simulink model "FullDuplex_UDP"  (R2017a)
settings: Solver=FixedStepDiscrete  StartTime=0.0  StopTime=10.0  FixedStep=0.0002  RelTol=1e-3
libraries: stellaris_lp_lib x20, simulink x4, xpcutilitieslib x2, dspswit3 x2
settings Model: ExtModeTrigDuration=8  Creator=peselnikmg  LastModifiedBy=Rorro
settings DataIOCC: LimitDataPoints=on  SaveFormat=Array  SignalLoggingSaveFormat=ModelDataLogs  ReturnWorkspaceOutputs=on
settings OptimizationCC: UseDivisionForNetSlopeComputation=on  UseFloatMulNetSlope=on  DefaultUnderspecifiedDataType=single  UseSpecifiedMinMax=on  PassReuseOutputArgsAs=Individual arguments  ExpressionDepthLimit=2147483647  ZeroExternalMemoryAtStartup=off  NoFixptDivByZeroProtection=on  EfficientFloat2IntCast=on  LifeSpan=inf  MaxStackSize=64  OptimizeBlockOrder=speed
settings DebuggingCC: ReadBeforeWriteMsg=DisableAll  WriteAfterWriteMsg=DisableAll  WriteAfterReadMsg=DisableAll  MultiTaskDSMMsg=none  IntegerOverflowMsg=error  ParameterTunabilityLossMsg=error  AssertControl=DisableAll  StateNameClashWarn=warning  NonBusSignalsTreatedAsBus=error  SFInvalidInputDataAccessInChartInitDiag=error  SFTransitionOutsideNaturalParentDiag=error  SFUnreachableExecutionPathDiag=error  SFUndirectedBroadcastEventsDiag=error  SFExecutionAtInitializationDiag=none  IntegerSaturationMsg=error
settings HardwareCC: ProdBitPerPointer=32  ProdBitPerSizeT=32  ProdBitPerPtrDiffT=32  ProdLargestAtomicInteger=Long  ProdLargestAtomicFloat=Double  ProdWordSize=32  ProdHWDeviceType=ARM Compatible->ARM Cortex
settings ModelReferenceCC: UpdateModelReferenceTargets=IfOutOfDate  PropagateSignalLabelsOutOfModel=off
settings SFSimCC: SFSimEcho=off  MATLABDynamicMemAlloc=off
settings RTWCC: SystemTargetFile=ert.tlc  HardwareBoard=Tiva TM4C123G Launchpad  TLCOptions=-aInlineSetEventsForThisBaseRateFcn=TLC_FALSE -aSuppressMultiTaskScheduler=TLC_FALSE -aRateBasedStepFcn=1  TemplateMakefile=ert_default_tmf  Description=Embedded Coder  GenerateReport=on  RTWVerbose=off  Toolchain=Texas Instruments Code Composer Studio (Tiva)  IncludeHyperlinkInReport=on  LaunchReport=on  GenerateTraceInfo=on  GenerateTraceReport=on  GenerateTraceReportSl=on  GenerateTraceReportSf=on  GenerateTraceReportEml=on
settings CodeAppCC: ForceParamTrailComments=on  IgnoreCustomStorageClasses=off  OperatorAnnotations=on  SimulinkDataObjDesc=on  SFDataObjDesc=on  MATLABFcnDesc=on  CustomSymbolStrType=$N$R$M  InsertBlockDesc=on  MATLABSourceComments=on  EnableCustomComments=on  ReqsInCode=on
settings ERTTargetCC: UtilityFuncGeneration=Shared location  CombineSignalStateStructs=on  SuppressErrorStatus=on  SupportNonFinite=off  ParenthesesLevel=Maximum  CastingMode=Standards  EnableSignedLeftShifts=off  EnableSignedRightShifts=off
settings ConfigComp: CovMetricSettings=dw  CovHtmlReporting=on  CovSaveCumulativeToWorkspaceVar=on  CovSaveSingleToWorkspaceVar=on  CovExternalEMLEnable=off

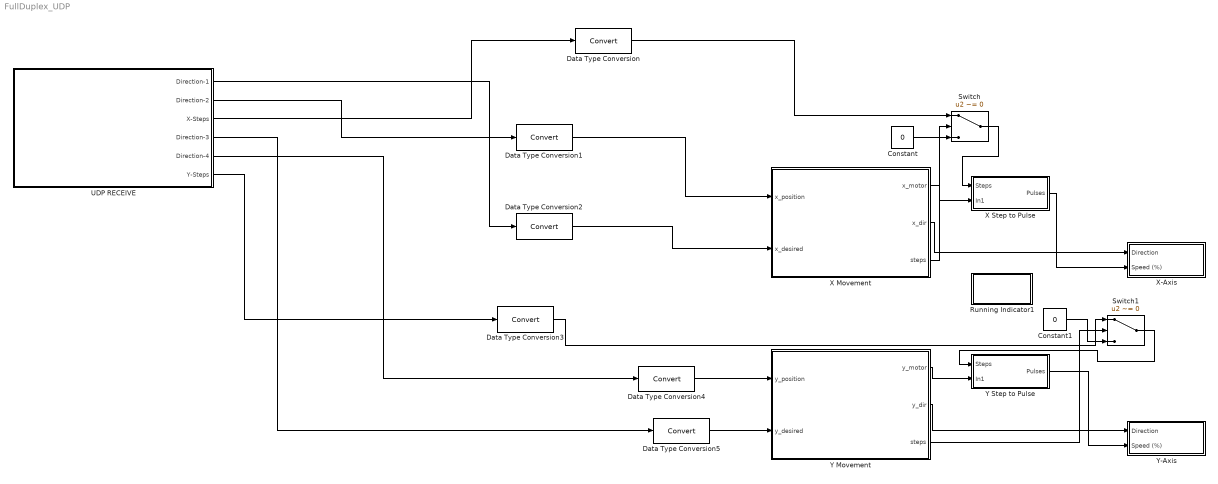
== system FullDuplex_UDP ==
  Constant : Constant  Value=0
  Constant1 : Constant  Value=0
  Data Type Conversion{,1..5} (6 alike) : DataTypeConversion
  Running Indicator1 : Subsystem
  Switch : Switch  Criteria=u2 ~= 0
  Switch1 : Switch  Criteria=u2 ~= 0
  UDP RECEIVE : Subsystem
  X Movement : Stateflow chart  TreatAsAtomicUnit=on
  X Step to Pulse : Subsystem  TreatAsAtomicUnit=on
  X-Axis : Subsystem
  Y Movement : Stateflow chart  TreatAsAtomicUnit=on
  Y Step to Pulse : Subsystem  TreatAsAtomicUnit=on
  Y-Axis : Subsystem
  wires:
  UDP RECEIVE/3(X-Steps) -> Data Type Conversion/1
  Data Type Conversion2/1 -> X Movement/2(x_desired)
  Data Type Conversion1/1 -> X Movement/1(x_position)
  UDP RECEIVE/1("Direction-1 ") -> Data Type Conversion2/1
  UDP RECEIVE/2("Direction-2 ") -> Data Type Conversion1/1
  Y Movement/2(y_dir) -> Y-Axis/1(Direction)
  Y Step to Pulse/1(Pulses) -> Y-Axis/2(Speed (%))
  X Movement/2(x_dir) -> X-Axis/1(Direction)
  Y Movement/1(y_motor) -> Y Step to Pulse/2(In1)
  X Movement/1(x_motor) -> X Step to Pulse/2(In1)
  X Step to Pulse/1(Pulses) -> X-Axis/2(Speed (%))
  UDP RECEIVE/4("Direction-3 ") -> Data Type Conversion5/1
  Data Type Conversion5/1 -> Y Movement/2(y_desired)
  UDP RECEIVE/5("Direction-4 ") -> Data Type Conversion4/1
  Data Type Conversion4/1 -> Y Movement/1(y_position)
  UDP RECEIVE/6(Y-Steps) -> Data Type Conversion3/1
  Data Type Conversion/1 -> Switch/1
  Constant/1 -> Switch/3
  X Movement/3(steps) -> Switch/2
  Switch/1 -> X Step to Pulse/1(Steps)
  Y Movement/3(steps) -> Switch1/2
  Constant1/1 -> Switch1/3
  Switch1/1 -> Y Step to Pulse/1(Steps)
  Data Type Conversion3/1 -> Switch1/1

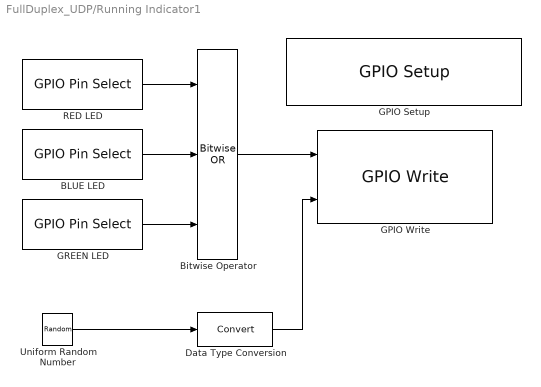
== system FullDuplex_UDP/Running Indicator1 ==
  BLUE LED : stellaris_lp_lib/GPIO/GPIO Pin Select  GPIO_PIN_X=GPIO_PIN_2
      settings: SourceProductName=Run on Stellaris LaunchPad
  Bitwise Operator : simulink/Logic and Bit Operations/Bitwise Operator  logicop=OR  UseBitMask=off  NumInputPorts=3  BitMask=bin2dec('11011001')  BitMaskRealWorld=Stored Integer
  Data Type Conversion : DataTypeConversion
  GPIO Setup : stellaris_lp_lib/GPIO/GPIO Setup  GPIO_PORTX_BASE=GPIO_PORTF_BASE  PinsOutput_0=Input  PinsOutput_1=Output  PinsOutput_2=Output  PinsOutput_3=Output  PinsOutput_4=Input  PinsOutput_5=Input  PinsOutput_6=Input  PinsOutput_7=Input
      settings: SourceProductName=Run on Stellaris LaunchPad
  GPIO Write : stellaris_lp_lib/GPIO/GPIO Write  GPIO_PORTX_BASE=GPIO_PORTF_BASE  SampleTime=-1
      settings: SourceProductName=Run on Stellaris LaunchPad
  GREEN LED : stellaris_lp_lib/GPIO/GPIO Pin Select  GPIO_PIN_X=GPIO_PIN_3
      settings: SourceProductName=Run on Stellaris LaunchPad
  RED LED : stellaris_lp_lib/GPIO/GPIO Pin Select  GPIO_PIN_X=GPIO_PIN_1
      settings: SourceProductName=Run on Stellaris LaunchPad
  Uniform Random Number : UniformRandomNumber  Minimum=0  Maximum=2  SampleTime=0.2
  wires:
  BLUE LED/1 -> Bitwise Operator/2
  RED LED/1 -> Bitwise Operator/1
  GREEN LED/1 -> Bitwise Operator/3
  Bitwise Operator/1 -> GPIO Write/1
  Uniform Random Number/1 -> Data Type Conversion/1
  Data Type Conversion/1 -> GPIO Write/2

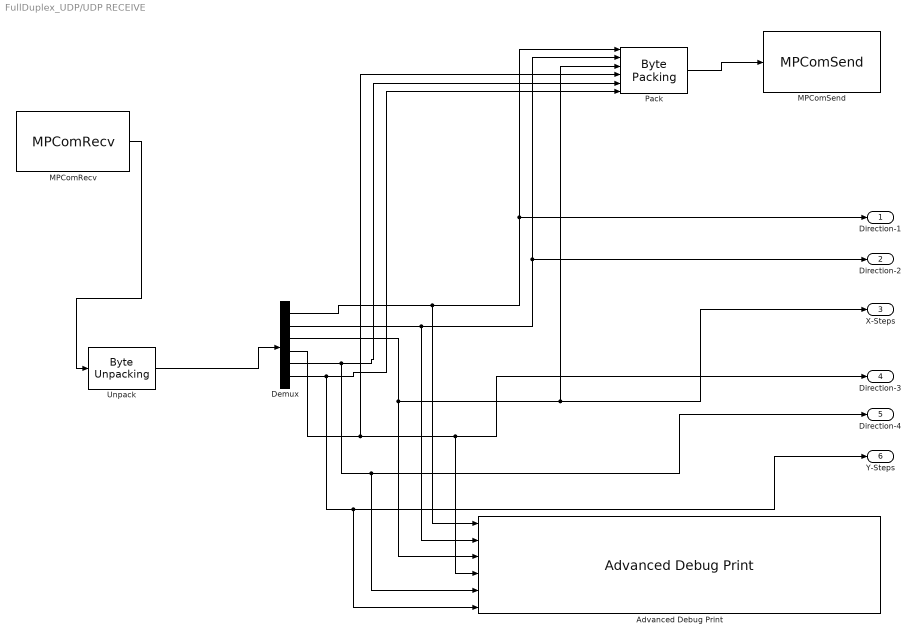
== system FullDuplex_UDP/UDP RECEIVE ==
  Advanced Debug Print : stellaris_lp_lib/Debug/Advanced Debug Print  types={'single','single','single','single','single','single'}  fmt='X: %hf %hf %hf\r\n'  sample_time=1
      settings: SourceProductName=Run on Stellaris LaunchPad
  Demux : Demux  Outputs=6
  MPComRecv : stellaris_lp_lib/Communication/MPComRecv  vport=2  pack_size=24  sample_time=-1
      settings: SourceProductName=Run on Stellaris LaunchPad
  MPComSend : stellaris_lp_lib/Communication/MPComSend  vport=3  pack_size=24  sample_time=-1
      settings: SourceProductName=Run on Stellaris LaunchPad
  Pack : xpcutilitieslib/Byte Packing   MaskPackedDataType=uint8  MaskUnpackedDataTypes={'single','single','single','single','single','single'}  MaskAlignment=1
  Unpack : xpcutilitieslib/Byte Unpacking   MaskUnpackedDataTypes={['single']}  MaskUnpackedDataSizes={[1,6]}  MaskAlignment=1
      settings: SourceProductName=Simulink Real-Time  SourceProductBaseCode=XP
  "Direction-1 " : Outport
  "Direction-2 " : Outport  Port=2
  X-Steps : Outport  Port=3
  "Direction-3 " : Outport  Port=4
  "Direction-4 " : Outport  Port=5
  Y-Steps : Outport  Port=6
  wires:
  Demux/1 -> Advanced Debug Print/1, "Direction-1 "/1, Pack/1
  Demux/2 -> Advanced Debug Print/2, "Direction-2 "/1, Pack/2
  Pack/1 -> MPComSend/1
  MPComRecv/1 -> Unpack/1
  Unpack/1 -> Demux/1
  Demux/3 -> Pack/3, X-Steps/1, Advanced Debug Print/3
  Demux/4 -> "Direction-3 "/1, Advanced Debug Print/4, Pack/4
  Demux/5 -> Pack/5, "Direction-4 "/1, Advanced Debug Print/5
  Demux/6 -> Pack/6, Y-Steps/1, Advanced Debug Print/6

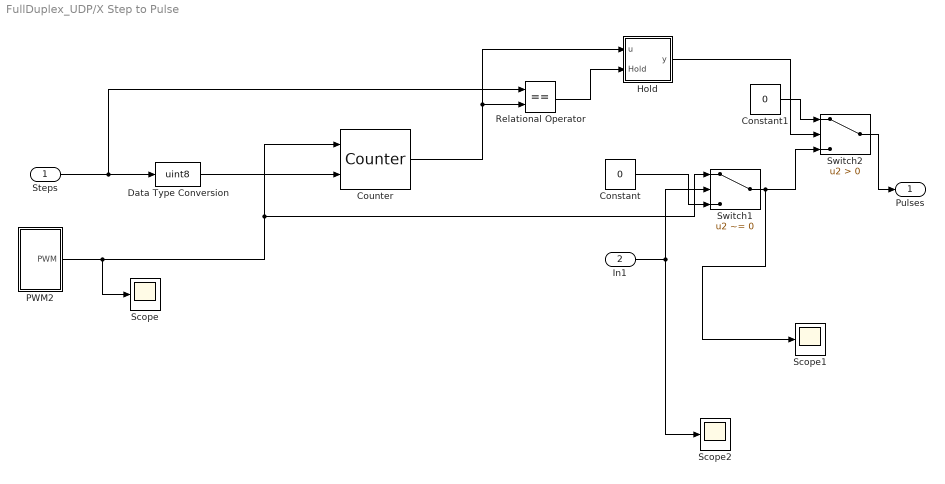
== system FullDuplex_UDP/X Step to Pulse ==
  Steps : Inport
  In1 : Inport  Port=2
  Constant : Constant  Value=0  OutDataTypeStr=single
  Constant1 : Constant  Value=0  OutDataTypeStr=single
  Counter : dspswit3/Counter  Direction=Up  CountEvent=Rising edge  CounterSize=Specify via input port  MaxCount=255  InitialCount=0  Output=Count  HitValue=2  ResetInput=off  SamplesPerFrame=1  Ts=1  CntDtype=single  HitDtype=Logical
  Data Type Conversion : DataTypeConversion  OutDataTypeStr=uint8
  Hold : Subsystem  TreatAsAtomicUnit=on
  PWM2 : Subsystem
  Relational Operator : RelationalOperator  Operator===  OutDataTypeStr=boolean  RndMeth=Simplest
  Scope : Scope
  Scope1 : Scope
  Scope2 : Scope
  Switch1 : Switch  Criteria=u2 ~= 0
  Switch2 : Switch  Criteria=u2 > Threshold
  Pulses : Outport
  wires:
  Steps/1 -> Relational Operator/1, Data Type Conversion/1
  Data Type Conversion/1 -> Counter/2
  Relational Operator/1 -> Hold/2(Hold)
  Switch1/1 -> Scope1/1, Switch2/3
  Counter/1 -> Hold/1(u), Relational Operator/2
  PWM2/1(PWM) -> Scope/1, Switch1/1, Counter/1
  In1/1 -> Scope2/1, Switch1/2
  Constant/1 -> Switch1/3
  Switch2/1 -> Pulses/1
  Constant1/1 -> Switch2/1
  Hold/1(y) -> Switch2/2

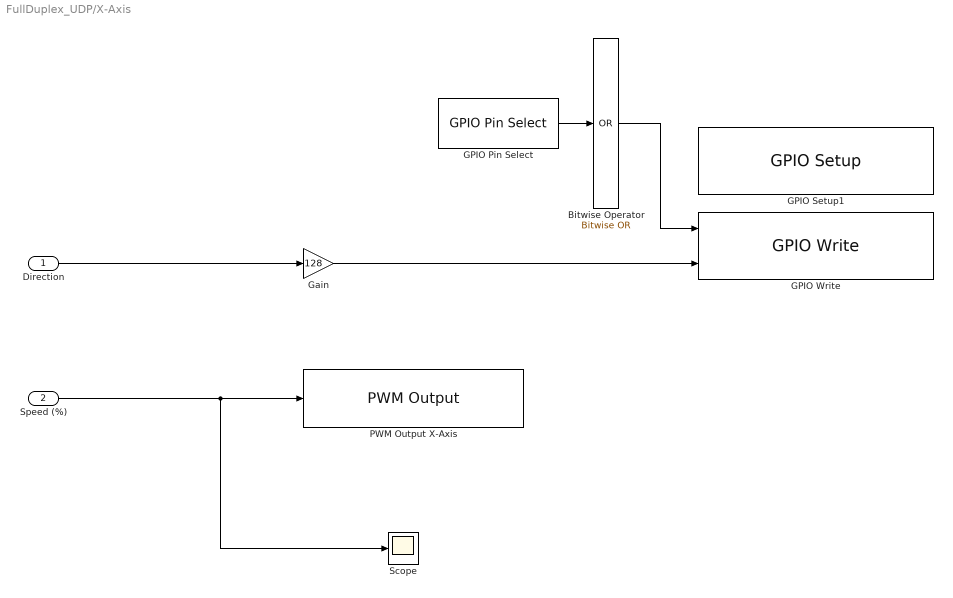
== system FullDuplex_UDP/X-Axis ==
  Direction : Inport  OutDataTypeStr=uint8
  Speed (%) : Inport  Port=2  OutDataTypeStr=single
  Bitwise Operator : simulink/Logic and Bit Operations/Bitwise Operator  logicop=OR  UseBitMask=off  BitMask=bin2dec('11011001')  BitMaskRealWorld=Real World Value
  GPIO Pin Select : stellaris_lp_lib/GPIO/GPIO Pin Select  GPIO_PIN_X=GPIO_PIN_7
      settings: SourceProductName=Run on Stellaris LaunchPad
  GPIO Setup1 : stellaris_lp_lib/GPIO/GPIO Setup  GPIO_PORTX_BASE=GPIO_PORTC_BASE  PinsOutput_0=Unused  PinsOutput_1=Unused  PinsOutput_2=Unused  PinsOutput_3=Unused  PinsOutput_4=Unused  PinsOutput_5=Unused  PinsOutput_6=Unused  PinsOutput_7=Output
      settings: SourceProductName=Run on Stellaris LaunchPad
  GPIO Write : stellaris_lp_lib/GPIO/GPIO Write  GPIO_PORTX_BASE=GPIO_PORTC_BASE  SampleTime=-1
      settings: SourceProductName=Run on Stellaris LaunchPad
  Gain : Gain  Gain=128  ParamDataTypeStr=uint8  OutDataTypeStr=uint8
  PWM Output X-Axis : stellaris_lp_lib/PWM/PWM Output  ch="1    PC4"  invert=off  freq=900  sample_time=-1
      settings: SourceProductName=Run on Stellaris LaunchPad
  Scope : Scope
  wires:
  Direction/1 -> Gain/1
  GPIO Pin Select/1 -> Bitwise Operator/1
  Bitwise Operator/1 -> GPIO Write/1
  Gain/1 -> GPIO Write/2
  Speed (%)/1 -> Scope/1, PWM Output X-Axis/1

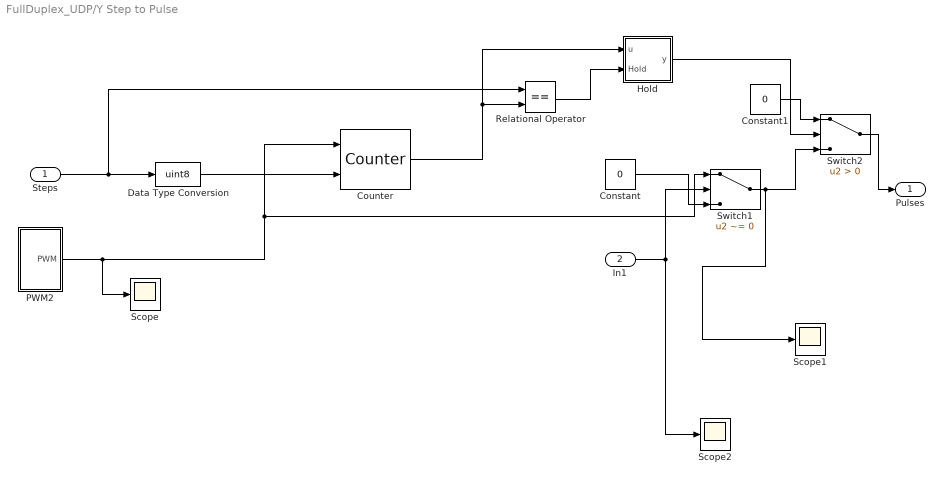
== system FullDuplex_UDP/Y Step to Pulse ==
  Steps : Inport
  In1 : Inport  Port=2
  Constant : Constant  Value=0  OutDataTypeStr=single
  Constant1 : Constant  Value=0  OutDataTypeStr=single
  Counter : dspswit3/Counter  Direction=Up  CountEvent=Rising edge  CounterSize=Specify via input port  MaxCount=255  InitialCount=0  Output=Count  HitValue=2  ResetInput=off  SamplesPerFrame=1  Ts=1  CntDtype=single  HitDtype=Logical
  Data Type Conversion : DataTypeConversion  OutDataTypeStr=uint8
  Hold : Subsystem  TreatAsAtomicUnit=on
  PWM2 : Subsystem
  Relational Operator : RelationalOperator  Operator===  OutDataTypeStr=boolean  RndMeth=Simplest
  Scope : Scope
  Scope1 : Scope
  Scope2 : Scope
  Switch1 : Switch  Criteria=u2 ~= 0
  Switch2 : Switch  Criteria=u2 > Threshold
  Pulses : Outport
  wires:
  Steps/1 -> Relational Operator/1, Data Type Conversion/1
  Data Type Conversion/1 -> Counter/2
  Relational Operator/1 -> Hold/2(Hold)
  Switch1/1 -> Scope1/1, Switch2/3
  Counter/1 -> Hold/1(u), Relational Operator/2
  PWM2/1(PWM) -> Scope/1, Switch1/1, Counter/1
  In1/1 -> Scope2/1, Switch1/2
  Constant/1 -> Switch1/3
  Switch2/1 -> Pulses/1
  Constant1/1 -> Switch2/1
  Hold/1(y) -> Switch2/2

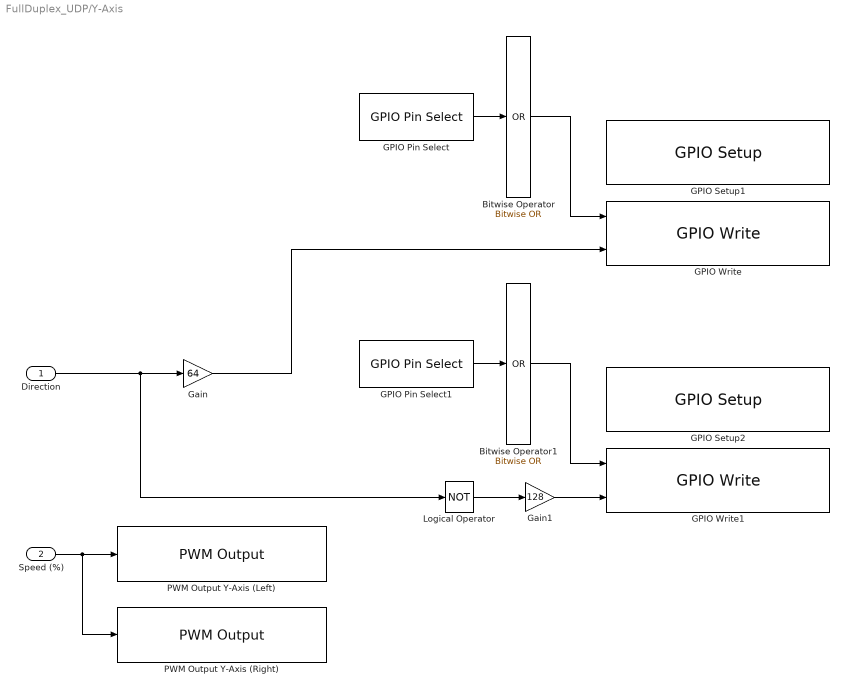
== system FullDuplex_UDP/Y-Axis ==
  Direction : Inport  OutDataTypeStr=uint8
  Speed (%) : Inport  Port=2  OutDataTypeStr=single
  Bitwise Operator : simulink/Logic and Bit Operations/Bitwise Operator  logicop=OR  UseBitMask=off  BitMask=bin2dec('11011001')  BitMaskRealWorld=Real World Value
  Bitwise Operator1 : simulink/Logic and Bit Operations/Bitwise Operator  logicop=OR  UseBitMask=off  BitMask=bin2dec('11011001')  BitMaskRealWorld=Real World Value
  GPIO Pin Select : stellaris_lp_lib/GPIO/GPIO Pin Select  GPIO_PIN_X=GPIO_PIN_6
      settings: SourceProductName=Run on Stellaris LaunchPad
  GPIO Pin Select1 : stellaris_lp_lib/GPIO/GPIO Pin Select  GPIO_PIN_X=GPIO_PIN_7
      settings: SourceProductName=Run on Stellaris LaunchPad
  GPIO Setup1 : stellaris_lp_lib/GPIO/GPIO Setup  GPIO_PORTX_BASE=GPIO_PORTD_BASE  PinsOutput_0=Unused  PinsOutput_1=Unused  PinsOutput_2=Unused  PinsOutput_3=Unused  PinsOutput_4=Unused  PinsOutput_5=Unused  PinsOutput_6=Output  PinsOutput_7=Unused
      settings: SourceProductName=Run on Stellaris LaunchPad
  GPIO Setup2 : stellaris_lp_lib/GPIO/GPIO Setup  GPIO_PORTX_BASE=GPIO_PORTD_BASE  PinsOutput_0=Unused  PinsOutput_1=Unused  PinsOutput_2=Unused  PinsOutput_3=Unused  PinsOutput_4=Unused  PinsOutput_5=Unused  PinsOutput_6=Unused  PinsOutput_7=Output
      settings: SourceProductName=Run on Stellaris LaunchPad
  GPIO Write : stellaris_lp_lib/GPIO/GPIO Write  GPIO_PORTX_BASE=GPIO_PORTD_BASE  SampleTime=-1
      settings: SourceProductName=Run on Stellaris LaunchPad
  GPIO Write1 : stellaris_lp_lib/GPIO/GPIO Write  GPIO_PORTX_BASE=GPIO_PORTD_BASE  SampleTime=-1
      settings: SourceProductName=Run on Stellaris LaunchPad
  Gain : Gain  Gain=64  ParamDataTypeStr=uint8  OutDataTypeStr=uint8
  Gain1 : Gain  Gain=128  OutDataTypeStr=uint8
  Logical Operator : Logic  Operator=NOT  AllPortsSameDT=off  OutDataTypeStr=boolean
  PWM Output Y-Axis (Left) : stellaris_lp_lib/PWM/PWM Output  ch="2    PC5"  invert=off  freq=900  sample_time=-1
      settings: SourceProductName=Run on Stellaris LaunchPad
  PWM Output Y-Axis (Right) : stellaris_lp_lib/PWM/PWM Output  ch="3    PC6"  invert=off  freq=900  sample_time=-1
      settings: SourceProductName=Run on Stellaris LaunchPad
  wires:
  Gain1/1 -> GPIO Write1/2
  Gain/1 -> GPIO Write/2
  Bitwise Operator1/1 -> GPIO Write1/1
  GPIO Pin Select1/1 -> Bitwise Operator1/1
  Speed (%)/1 -> PWM Output Y-Axis (Left)/1, PWM Output Y-Axis (Right)/1
  Logical Operator/1 -> Gain1/1
  Bitwise Operator/1 -> GPIO Write/1
  GPIO Pin Select/1 -> Bitwise Operator/1
  Direction/1 -> Logical Operator/1, Gain/1

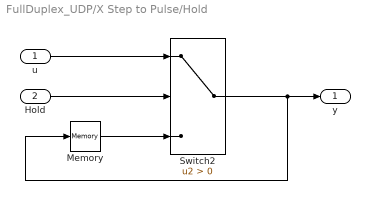
== system FullDuplex_UDP/X Step to Pulse/Hold ==
  u : Inport  OutDataTypeStr=single
  Hold : Inport  Port=2  OutDataTypeStr=boolean
  Memory : Memory
  Switch2 : Switch  Criteria=u2 > Threshold  OutDataTypeStr=single
  y : Outport  OutDataTypeStr=single
  wires:
  u/1 -> Switch2/1
  Switch2/1 -> Memory/1, y/1
  Memory/1 -> Switch2/3
  Hold/1 -> Switch2/2

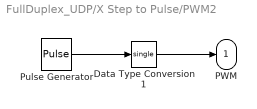
== system FullDuplex_UDP/X Step to Pulse/PWM2 ==
  Data Type Conversion1 : DataTypeConversion  OutDataTypeStr=single
  Pulse Generator : DiscretePulseGenerator  PulseType=Time based  Amplitude=50  Period=.1  PulseWidth=98
  PWM : Outport
  wires:
  Pulse Generator/1 -> Data Type Conversion1/1
  Data Type Conversion1/1 -> PWM/1

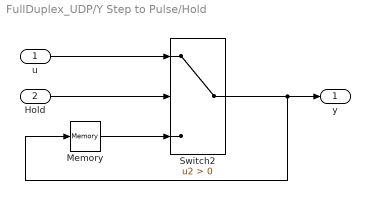
== system FullDuplex_UDP/Y Step to Pulse/Hold ==
  u : Inport  OutDataTypeStr=single
  Hold : Inport  Port=2  OutDataTypeStr=boolean
  Memory : Memory
  Switch2 : Switch  Criteria=u2 > Threshold  OutDataTypeStr=single
  y : Outport  OutDataTypeStr=single
  wires:
  u/1 -> Switch2/1
  Switch2/1 -> Memory/1, y/1
  Memory/1 -> Switch2/3
  Hold/1 -> Switch2/2

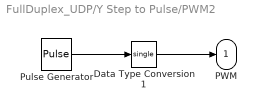
== system FullDuplex_UDP/Y Step to Pulse/PWM2 ==
  Data Type Conversion1 : DataTypeConversion  OutDataTypeStr=single
  Pulse Generator : DiscretePulseGenerator  PulseType=Time based  Amplitude=50  Period=.1  PulseWidth=98
  PWM : Outport
  wires:
  Pulse Generator/1 -> Data Type Conversion1/1
  Data Type Conversion1/1 -> PWM/1

== stateflow chart FullDuplex_UDP/X Movement ==
  state Motor_Moving_CCW1
    entry:
    steps = 1;
    x_dir = 0;
    x_motor = 1;
    exit:
    x_motor = 0;
    steps = 0;
  state Motor_Still
    entry:
    steps = 1;
    x_motor = 0;
    exit:
    steps = 0;
  state Motor_Moving_CW
    entry:
    steps = 1;
    x_dir = 1;
    x_motor = 1;
    exit:
    x_motor = 0;
    steps = 0;
  (default) -> Motor_Still
  Motor_Still -> Motor_Moving_CCW1 [order 1] : [x_position < x_desired]
  Motor_Moving_CCW1 -> Motor_Still [order 1] : [x_position == x_desired]
  Motor_Moving_CW -> Motor_Still [order 1] : [x_position == x_desired]
  Motor_Still -> Motor_Moving_CW [order 2] : [x_position > x_desired]
  Motor_Moving_CCW1 -> Motor_Moving_CW [order 2] : [x_position > x_desired]
  Motor_Moving_CW -> Motor_Moving_CCW1 [order 2] : [x_position < x_desired]
  data: x_position input; x_desired input; x_motor output uint8; x_dir output uint8; steps output single

== stateflow chart FullDuplex_UDP/Y Movement ==
  state Motor_Still
    entry:
    steps = 1;
    y_motor = 0;
  state Motor_Moving_CCW1
    entry:
    steps = 1;
    y_dir = 0;
    y_motor = 1;
    exit:
    y_motor = 0;
    steps = 0;
  state Motor_Moving_CW
    entry:
    steps = 1;
    y_dir = 1;
    y_motor = 1;
    exit:
    y_motor = 0;
    steps = 0;
  (default) -> Motor_Still
  Motor_Still -> Motor_Moving_CCW1 [order 1] : [y_position < y_desired]
  Motor_Moving_CCW1 -> Motor_Still [order 1] : [y_position == y_desired]
  Motor_Moving_CW -> Motor_Still [order 1] : [y_position == y_desired]
  Motor_Still -> Motor_Moving_CW [order 2] : [y_position > y_desired]
  Motor_Moving_CW -> Motor_Moving_CCW1 [order 2] : [y_position < y_desired]
  Motor_Moving_CCW1 -> Motor_Moving_CW [order 2] : [y_position > y_desired]
  data: y_position input; y_desired input; y_motor output uint8; y_dir output uint8; steps output single
